simulink model "vibeNotch"  (R2014a)
settings: Solver=ode45  StartTime=0.0  StopTime=10.0  RelTol=1e-3
undefined symbols (not defined in the file or in its folder): loopNotchQA
settings Model: Creator=s220385  LastModifiedBy=s220385

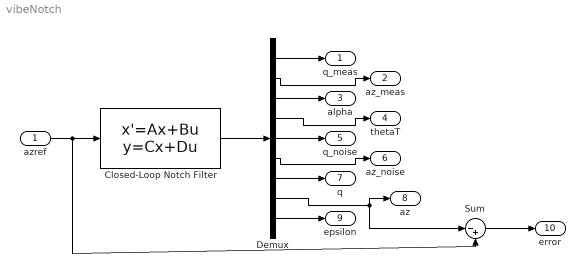
== system vibeNotch ==
  azref : Inport
  Closed-Loop Notch Filter : StateSpace  A=loopNotchQA.a  B=loopNotchQA.b  C=loopNotchQA.c  D=loopNotchQA.d  X0=0
  Demux : Demux  Outputs=9
  Sum : Sum  Inputs=|-+
  q_meas : Outport
  az_meas : Outport  Port=2
  alpha : Outport  Port=3
  thetaT : Outport  Port=4
  q_noise : Outport  Port=5
  az_noise : Outport  Port=6
  q : Outport  Port=7
  az : Outport  Port=8
  epsilon : Outport  Port=9
  error : Outport  Port=10
  wires:
  Closed-Loop Notch Filter/1 -> Demux/1
  Demux/9 -> epsilon/1
  Demux/5 -> q_noise/1
  Demux/3 -> alpha/1
  Demux/7 -> q/1
  Demux/1 -> q_meas/1
  Demux/4 -> thetaT/1
  Demux/6 -> az_noise/1
  Demux/2 -> az_meas/1
  Demux/8 -> az/1, Sum/1
  azref/1 -> Sum/2, Closed-Loop Notch Filter/1
  Sum/1 -> error/1
